simulink model "multiple_equations_simulation"  (R2024a)
settings: Solver=VariableStepAuto  StartTime=0.0  StopTime=10.0  RelTol=1e-3
settings Model: Creator=deban  LastModifiedBy=deban

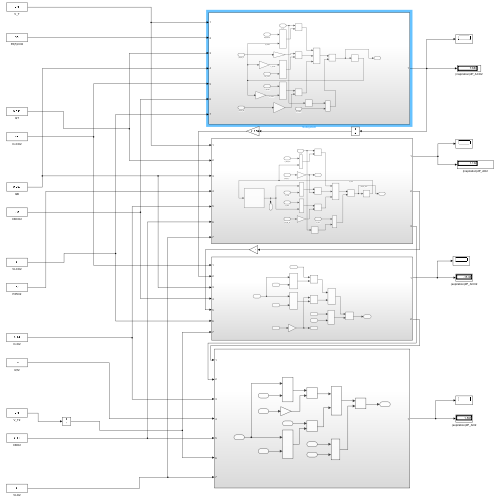
[thumbnail: Simulink's stored preview of the top-level diagram]
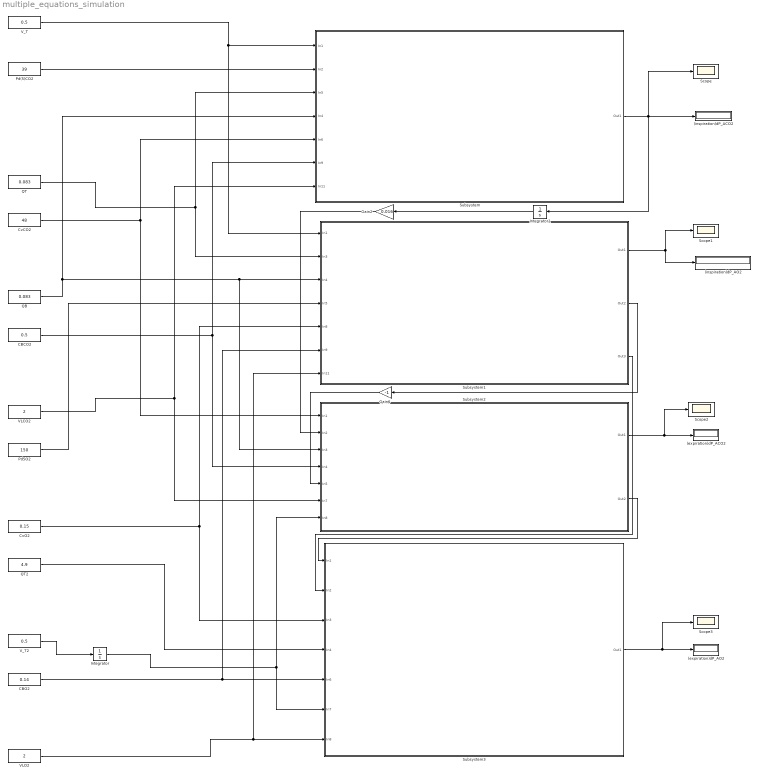
== system multiple_equations_simulation ==
  (expiration)dP_ACO2 : Display
  (expiration)dP_AO2 : Display
  (inspiration)dP_ACO2 : Display
  (inspiration)dP_AO2 : Display
  CBCO2 : Constant  Value=0.5
  CBO2 : Constant  Value=0.14
  CvCO2 : Constant  Value=48
  CvO2 : Constant  Value=0.15
  Gain2 : Gain  Gain=0.016
  Gain6 : Gain  Gain=-1
  Integrator : Integrator  InitialCondition=35
  Integrator1 : Integrator  InitialCondition=40
  Pd(5)CO2 : Constant  Value=39
  Pd5O2 : Constant  Value=150
  QB : Constant  Value=0.083
  QT : Constant  Value=0.083
  QT2 : Constant  Value=4.9
  Scope{,1..3} (4 alike) : Scope
  Subsystem : Subsystem
  Subsystem1 : Subsystem
  Subsystem2 : Subsystem
  Subsystem3 : Subsystem
  VLCO2 : Constant  Value=2
  VLO2 : Constant  Value=2
  V_T : Constant  Value=0.5
  V_T2 : Constant  Value=0.5
  wires:
  V_T/1 -> Subsystem1/1(In1), Subsystem/1(In1)
  QT/1 -> Subsystem1/2(In3), Subsystem/3(In5)
  CvCO2/1 -> Subsystem/5(In6), Subsystem2/1(In1)
  CBCO2/1 -> Subsystem2/4(In4), Subsystem/6(In9)
  VLCO2/1 -> Subsystem2/6(In7), Subsystem/7(In11)
  CvO2/1 -> Subsystem1/5(In8), Subsystem3/3(In3)
  CBO2/1 -> Subsystem1/6(In9), Subsystem3/5(In6)
  VLO2/1 -> Subsystem1/7(In11), Subsystem3/7(In8)
  V_T2/1 -> Integrator/1
  Pd(5)CO2/1 -> Subsystem/2(In2)
  Pd5O2/1 -> Subsystem1/4(In5)
  Subsystem1/1(Out1) -> (inspiration)dP_AO2/1, Scope1/1
  Subsystem1/2(Out2) -> Gain6/1
  Gain6/1 -> Subsystem2/5(In5)
  Subsystem2/1(Out1) -> Scope2/1, (expiration)dP_ACO2/1
  Subsystem2/2(Out2) -> Subsystem3/1(In1)
  QT2/1 -> Subsystem3/4(In4)
  Subsystem3/1(Out1) -> Scope3/1, (expiration)dP_AO2/1
  Subsystem/1(Out1) -> Integrator1/1, (inspiration)dP_ACO2/1, Scope/1
  Integrator/1 -> Subsystem2/7(In8), Subsystem3/6(In7)
  QB/1 -> Subsystem/4(In4), Subsystem2/3(In3), Subsystem1/3(In4)
  Integrator1/1 -> Gain2/1
  Gain2/1 -> Subsystem2/2(In2)
  Subsystem1/3(Out3) -> Subsystem3/2(In2)

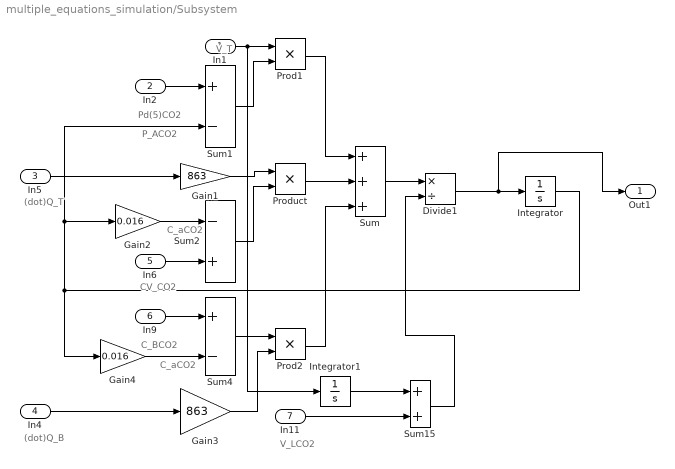
== system multiple_equations_simulation/Subsystem ==
  note: (dot)Q_B
  note: P_ACO2
  note: V_LCO2
  note: C_aCO2
  note: C_BCO2
  note: C_aCO2
  note: CV_CO2
  note: (dot)Q_T
  note: Pd(5)CO2
  note: V_T
  In1 : Inport
  In2 : Inport  Port=2
  In5 : Inport  Port=3
  In4 : Inport  Port=4
  In6 : Inport  Port=5
  In9 : Inport  Port=6
  In11 : Inport  Port=7
  Divide1 : Product  Inputs=*/
  Gain1 : Gain  Gain=863
  Gain2 : Gain  Gain=0.016
  Gain3 : Gain  Gain=863
  Gain4 : Gain  Gain=0.016
  Integrator : Integrator  InitialCondition=40
  Integrator1 : Integrator  InitialCondition=2.8
  Prod1 : Product
  Prod2 : Product
  Product : Product
  Sum : Sum  Inputs=+++
  Sum1 : Sum  Inputs=+-
  Sum15 : Sum
  Sum2 : Sum  Inputs=-+
  Sum4 : Sum  Inputs=+-
  Out1 : Outport
  wires:
  In6/1 -> Sum2/2
  Sum15/1 -> Divide1/2
  Sum2/1 -> Product/2
  Gain1/1 -> Product/1
  In5/1 -> Gain1/1
  Integrator/1 -> Gain4/1, Gain2/1, Sum1/2
  In9/1 -> Sum4/1
  In1/1 -> Integrator1/1, Prod1/1
  Sum1/1 -> Prod1/2
  Sum4/1 -> Prod2/1
  Gain3/1 -> Prod2/2
  Prod2/1 -> Sum/3
  Prod1/1 -> Sum/1
  Product/1 -> Sum/2
  In11/1 -> Sum15/2
  Sum/1 -> Divide1/1
  Divide1/1 -> Out1/1, Integrator/1
  Integrator1/1 -> Sum15/1
  In4/1 -> Gain3/1
  Gain2/1 -> Sum2/1
  Gain4/1 -> Sum4/2
  In2/1 -> Sum1/1

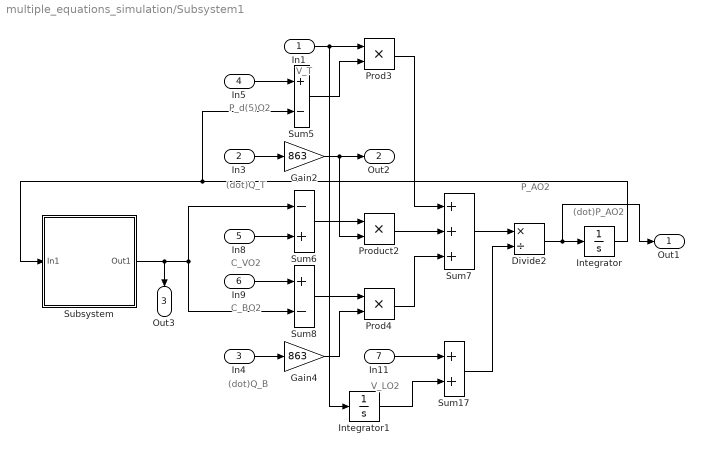
== system multiple_equations_simulation/Subsystem1 ==
  note: P_AO2
  note: (dot)P_AO2
  note: V_LO2
  note: (dot)Q_B
  note: C_BO2
  note: C_VO2
  note: (dot)Q_T
  note: P_d(5)O2
  note: V_T
  In1 : Inport
  In3 : Inport  Port=2
  In4 : Inport  Port=3
  In5 : Inport  Port=4
  In8 : Inport  Port=5
  In9 : Inport  Port=6
  In11 : Inport  Port=7
  Divide2 : Product  Inputs=*/
  Gain2 : Gain  Gain=863
  Gain4 : Gain  Gain=863
  Integrator : Integrator  InitialCondition=40
  Integrator1 : Integrator  InitialCondition=35
  Prod3 : Product
  Prod4 : Product
  Product2 : Product
  Subsystem : Subsystem
  Sum17 : Sum
  Sum5 : Sum  Inputs=+-
  Sum6 : Sum  Inputs=-+
  Sum7 : Sum  Inputs=+++
  Sum8 : Sum  Inputs=+-
  Out1 : Outport
  Out2 : Outport  Port=2
  Out3 : Outport  Port=3
  wires:
  In4/1 -> Gain4/1
  In9/1 -> Sum8/1
  In8/1 -> Sum6/2
  In11/1 -> Sum17/1
  In3/1 -> Gain2/1
  In5/1 -> Sum5/1
  In1/1 -> Integrator1/1, Prod3/1
  Sum6/1 -> Product2/1
  Sum5/1 -> Prod3/2
  Gain2/1 -> Product2/2, Out2/1
  Sum8/1 -> Prod4/1
  Gain4/1 -> Prod4/2
  Prod4/1 -> Sum7/3
  Prod3/1 -> Sum7/1
  Product2/1 -> Sum7/2
  Sum7/1 -> Divide2/1
  Sum17/1 -> Divide2/2
  Divide2/1 -> Out1/1, Integrator/1
  Integrator1/1 -> Sum17/2
  Integrator/1 -> Subsystem/1(In1), Sum5/2
  Subsystem/1(Out1) -> Out3/1, Sum6/1, Sum8/2

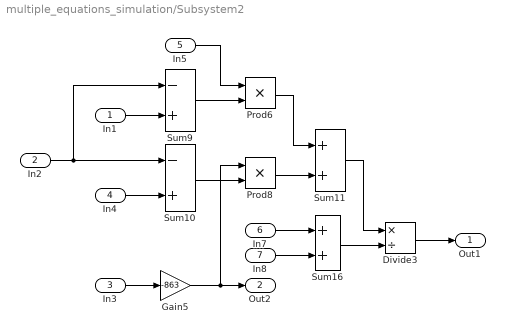
== system multiple_equations_simulation/Subsystem2 ==
  In1 : Inport
  In2 : Inport  Port=2
  In3 : Inport  Port=3
  In4 : Inport  Port=4
  In5 : Inport  Port=5
  In7 : Inport  Port=6
  In8 : Inport  Port=7
  Divide3 : Product  Inputs=*/
  Gain5 : Gain  Gain=-863
  Prod6 : Product
  Prod8 : Product
  Sum10 : Sum  Inputs=-+
  Sum11 : Sum
  Sum16 : Sum
  Sum9 : Sum  Inputs=-+
  Out1 : Outport
  Out2 : Outport  Port=2
  wires:
  In5/1 -> Prod6/1
  Prod8/1 -> Sum11/2
  In3/1 -> Gain5/1
  In4/1 -> Sum10/2
  In2/1 -> Sum10/1, Sum9/1
  In1/1 -> Sum9/2
  Sum9/1 -> Prod6/2
  Sum10/1 -> Prod8/2
  Gain5/1 -> Prod8/1, Out2/1
  Prod6/1 -> Sum11/1
  In7/1 -> Sum16/1
  In8/1 -> Sum16/2
  Sum11/1 -> Divide3/1
  Sum16/1 -> Divide3/2
  Divide3/1 -> Out1/1

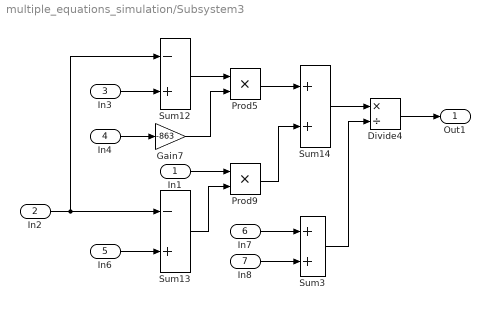
== system multiple_equations_simulation/Subsystem3 ==
  In1 : Inport
  In2 : Inport  Port=2
  In3 : Inport  Port=3
  In4 : Inport  Port=4
  In6 : Inport  Port=5
  In7 : Inport  Port=6
  In8 : Inport  Port=7
  Divide4 : Product  Inputs=*/
  Gain7 : Gain  Gain=-863
  Prod5 : Product
  Prod9 : Product
  Sum12 : Sum  Inputs=-+
  Sum13 : Sum  Inputs=-+
  Sum14 : Sum
  Sum3 : Sum
  Out1 : Outport
  wires:
  In1/1 -> Prod9/1
  Sum14/1 -> Divide4/1
  Sum13/1 -> Prod9/2
  In2/1 -> Sum13/1, Sum12/1
  Sum12/1 -> Prod5/1
  In6/1 -> Sum13/2
  In4/1 -> Gain7/1
  In3/1 -> Sum12/2
  Gain7/1 -> Prod5/2
  Prod5/1 -> Sum14/1
  Prod9/1 -> Sum14/2
  In7/1 -> Sum3/1
  In8/1 -> Sum3/2
  Sum3/1 -> Divide4/2
  Divide4/1 -> Out1/1

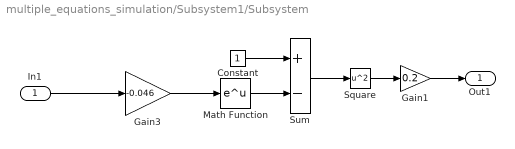
== system multiple_equations_simulation/Subsystem1/Subsystem ==
  In1 : Inport
  Constant : Constant
  Gain1 : Gain  Gain=0.2
  Gain3 : Gain  Gain=-0.046
  Math Function : Math
  Square : Math  Operator=square
  Sum : Sum  Inputs=+-
  Out1 : Outport
  wires:
  Square/1 -> Gain1/1
  Gain3/1 -> Math Function/1
  In1/1 -> Gain3/1
  Constant/1 -> Sum/1
  Gain1/1 -> Out1/1
  Math Function/1 -> Sum/2
  Sum/1 -> Square/1
